simulink model "cart_pend_simulation"  (R2020a)
settings: Solver=VariableStepAuto  StartTime=0.0  StopTime=150  RelTol=1e-3
values from neighbouring files (symbols this model uses):
  a = 1/(M+m)    (= 0.1)    [cart_pend_script.m]
  A1 = [-1 max(z1) ... (first row only)    [TS_modling_script.m]    (also in cart_pend_script.m = [0 1 0 0; -17.31 0 0 0; 0 0 0 1; 1.7312 0 0 0])
  A2 = [-1 max(z1) ... (first row only)    [TS_modling_script.m]    (also in cart_pend_script.m = [0 1 0 0; -14.32 0 0 0; 0 0 0 1; 0.716 0 0 0])
  B1 = [0; -0.1765; 0; 0.1176]    [cart_pend_script.m]
  B2 = [0; -0.1147; 0; 0.1081]    [cart_pend_script.m]
  C = [1 0 0 0; 0 0 1 0; 0 0 0 1]    [cart_pend_script.m]
  g = 9.81    [cart_pend_script.m]
  Gl = [4 0 -1.5; -14.31 0 -6; 0 2 1; 1.73 0 4]    [cart_pend_script.m]
  Gnl = [0.1176 0 0; 0.3529 0 -0.1765; 0 0.1176 0; 0 0 0.1176]    [cart_pend_script.m]
  KK1 = lqr(Abf1,B1,Q,R,N)    [cart_pend_script.m]
  l = 0.5    [cart_pend_script.m]
  m = 2    [cart_pend_script.m]
  uc = 0.005    [cart_pend_script.m]
  x0 = [-0.7;1]    [TS_modling_script.m]    (also in cart_pend_script.m = [0.6; 0; 0.1; 0])
settings Model: Creator=pc  LastModifiedBy=hp
settings SolverCC: ZeroCrossAlgorithm=Adaptive
settings DebuggingCC: IgnoredZcDiagnostic=none

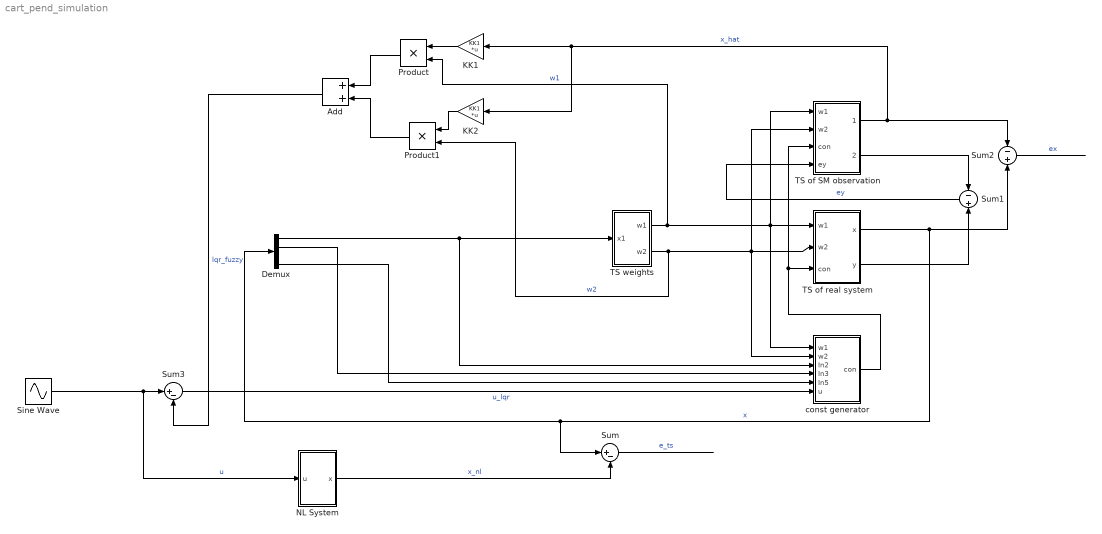
== system cart_pend_simulation ==
  Add : Sum
  Demux : Demux
  KK1 : Gain  Gain=KK1  Multiplication=Matrix(K*u)
  KK2 : Gain  Gain=KK1  Multiplication=Matrix(K*u)
  NL System : Subsystem
  Product : Product
  Product1 : Product
  Sine Wave : Sin  Amplitude=10  Frequency=5  SampleTime=0
  Sum : Sum  Inputs=|+-
  Sum1 : Sum  Inputs=-+
  Sum2 : Sum  Inputs=-+
  Sum3 : Sum  Inputs=|+-
  TS of SM observation : Subsystem
  TS of real system : Subsystem
  TS weights : Subsystem
  const generator : Subsystem
  wires:
  Demux/1 -> TS weights/1(x1), const generator/3(In2)
  TS weights/1(w1) -> Product/2, TS of SM observation/1(w1), const generator/1(w1), TS of real system/1(w1)  "w1"
  TS weights/2(w2) -> Product1/2, TS of SM observation/2(w2), const generator/2(w2), TS of real system/2(w2)  "w2"
  TS of real system/1(x) -> Sum/1, Demux/1, Sum2/2  "x"
  Demux/2 -> const generator/4(In3)
  Demux/4 -> const generator/5(In5)
  const generator/1(con) -> TS of SM observation/3(con), TS of real system/3(con)
  NL System/1(x) -> Sum/2  "x_nl"
  Sum/1 -> ?  "e_ts"
  Sum1/1 -> TS of SM observation/4(ey)  "ey"
  TS of SM observation/2(y_hat) -> Sum1/1
  TS of real system/2(y) -> Sum1/2
  TS of SM observation/1(x_hat) -> KK2/1, KK1/1, Sum2/1  "x_hat"
  Sum2/1 -> ?  "ex"
  Sine Wave/1 -> Sum3/1, NL System/1(u)  "u"
  Sum3/1 -> const generator/6(u)  "u_lqr"
  KK1/1 -> Product/1
  Product/1 -> Add/1
  KK2/1 -> Product1/1
  Product1/1 -> Add/2
  Add/1 -> Sum3/2  "lqr_fuzzy"

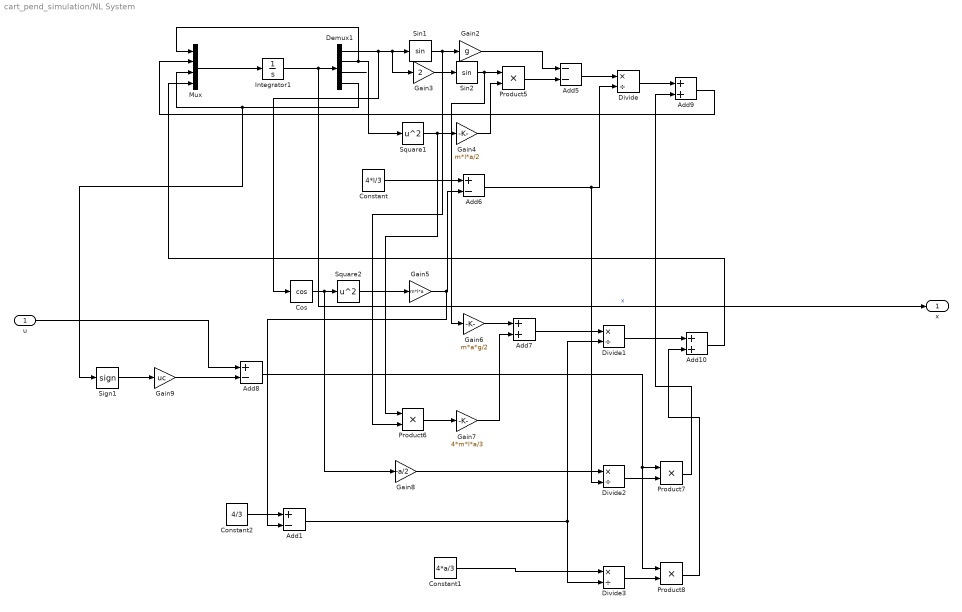
== system cart_pend_simulation/NL System ==
  u : Inport
  Add1 : Sum  Inputs=+-
  Add10 : Sum
  Add5 : Sum  Inputs=--
  Add6 : Sum  Inputs=+-
  Add7 : Sum
  Add8 : Sum  Inputs=+-
  Add9 : Sum
  Constant : Constant  Value=4*l/3
  Constant1 : Constant  Value=4*a/3
  Constant2 : Constant  Value=4/3
  Cos : Trigonometry  Operator=cos
  Demux1 : Demux
  Divide{,1..3} (4 alike) : Product  Inputs=*/
  Gain2 : Gain  Gain=g
  Gain3 : Gain  Gain=2
  Gain4 : Gain  Gain=m*l*a/2
  Gain5 : Gain  Gain=m*l*a
  Gain6 : Gain  Gain=m*a*g/2
  Gain7 : Gain  Gain=4*m*l*a/3
  Gain8 : Gain  Gain=-a/2
  Gain9 : Gain  Gain=uc
  Integrator1 : Integrator  InitialCondition=x0
  Mux : Mux
  Product{5..8} (4 alike) : Product
  Sign1 : Signum
  Sin1 : Trigonometry
  Sin2 : Trigonometry
  Square1 : Math  Operator=square  SaturateOnIntegerOverflow=on
  Square2 : Math  Operator=square  SaturateOnIntegerOverflow=on
  x : Outport
  wires:
  Add5/1 -> Divide/1
  Divide3/1 -> Product8/2
  Add9/1 -> Mux/2
  Add8/1 -> Product8/1, Product7/1
  Product5/1 -> Add5/2
  Square2/1 -> Gain5/1
  Demux1/4 -> Sign1/1, Mux/3
  Constant2/1 -> Add1/1
  Demux1/1 -> Cos/1, Gain3/1, Sin1/1
  Demux1/3 -> ?
  Add1/1 -> Divide1/2, Divide3/2
  Sin2/1 -> Gain6/1, Product5/1
  Add7/1 -> Divide1/1
  u/1 -> Add8/1
  Cos/1 -> Gain8/1, Square2/1
  Gain4/1 -> Product5/2
  Constant/1 -> Add6/1
  Divide1/1 -> Add10/1
  Gain5/1 -> Add1/2, Add6/2
  Gain9/1 -> Add8/2
  Product6/1 -> Gain7/1
  Divide2/1 -> Product7/2
  Gain8/1 -> Divide2/1
  Add6/1 -> Divide/2, Divide2/2
  Gain3/1 -> Sin2/1
  Sign1/1 -> Gain9/1
  Sin1/1 -> Product6/2, Gain2/1
  Square1/1 -> Product6/1, Gain4/1
  Gain2/1 -> Add5/1
  Product7/1 -> Add9/2
  Add10/1 -> Mux/4
  Product8/1 -> Add10/2
  Mux/1 -> Integrator1/1
  Demux1/2 -> Square1/1, Mux/1
  Gain7/1 -> Add7/2
  Integrator1/1 -> x/1, Demux1/1  "x"
  Divide/1 -> Add9/1
  Constant1/1 -> Divide3/1
  Gain6/1 -> Add7/1

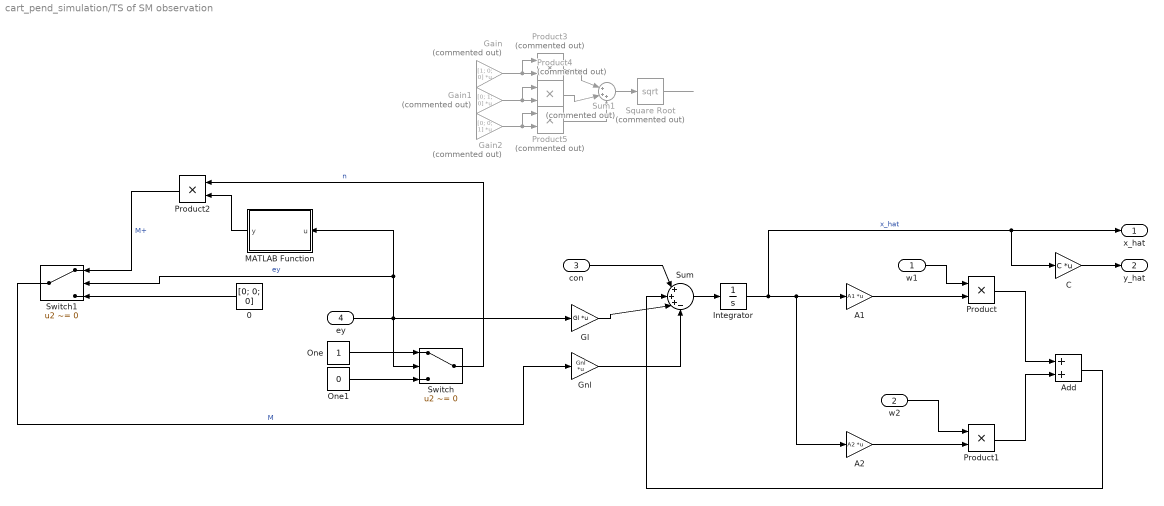
== system cart_pend_simulation/TS of SM observation ==
  w1 : Inport
  w2 : Inport  Port=2
  con : Inport  Port=3
  ey : Inport  Port=4
  0 : Constant  Value=[0; 0; 0]  VectorParams1D=off  OutDataTypeStr=Inherit: Inherit via back propagation
  A1 : Gain  Gain=A1  Multiplication=Matrix(K*u)
  A2 : Gain  Gain=A2  Multiplication=Matrix(K*u)
  Add : Sum
  C : Gain  Gain=C  Multiplication=Matrix(K*u)
  Gain : Gain  Commented=on  Gain=[1; 0; 0]  Multiplication=Matrix(K*u)
  Gain1 : Gain  Commented=on  Gain=[0; 1; 0]  Multiplication=Matrix(K*u)
  Gain2 : Gain  Commented=on  Gain=[0; 0; 1]  Multiplication=Matrix(K*u)
  Gl : Gain  Gain=Gl  Multiplication=Matrix(K*u)
  Gnl : Gain  Gain=Gnl  Multiplication=Matrix(K*u)
  Integrator : Integrator  InitialCondition=[0; 0; 0; 0]
  MATLAB Function : MATLAB Function  TreatAsAtomicUnit=on
  One : Constant  OutDataTypeStr=Inherit: Inherit via back propagation
  One1 : Constant  Value=0  OutDataTypeStr=Inherit: Inherit via back propagation
  Product : Product
  Product1 : Product
  Product2 : Product
  Product3 : Product  Commented=on
  Product4 : Product  Commented=on
  Product5 : Product  Commented=on
  Square Root : Sqrt  Commented=on  SaturateOnIntegerOverflow=on
  Sum : Sum  Inputs=|+++-
  Sum1 : Sum  Commented=on  Inputs=|+++
  Switch : Switch  Criteria=u2 ~= 0  ZeroCross=off
  Switch1 : Switch  Criteria=u2 ~= 0  ZeroCross=off
  x_hat : Outport
  y_hat : Outport  Port=2
  wires:
  Product/1 -> Add/1
  Integrator/1 -> C/1, x_hat/1, A2/1, A1/1  "x_hat"
  Add/1 -> Sum/2
  Sum/1 -> Integrator/1
  A1/1 -> Product/2
  A2/1 -> Product1/2
  Product1/1 -> Add/2
  w2/1 -> Product1/1
  w1/1 -> Product/1
  ey/1 -> Switch/2, Switch1/2, MATLAB Function/1(u), Gl/1  "ey"
  Gl/1 -> Sum/3
  Gnl/1 -> Sum/4
  C/1 -> y_hat/1
  One/1 -> Switch/1
  One1/1 -> Switch/3
  Switch1/1 -> Gnl/1  "M"
  MATLAB Function/1(y) -> Product2/2
  con/1 -> Sum/1
  Gain/1 -> Product3/1, Product3/2
  Gain1/1 -> Product4/1, Product4/2
  Gain2/1 -> Product5/1, Product5/2
  Product3/1 -> Sum1/1
  Product4/1 -> Sum1/2
  Product5/1 -> Sum1/3
  Sum1/1 -> Square Root/1
  Square Root/1 -> ?
  0/1 -> Switch1/3
  Product2/1 -> Switch1/1  "M+"
  Switch/1 -> Product2/1  "n"

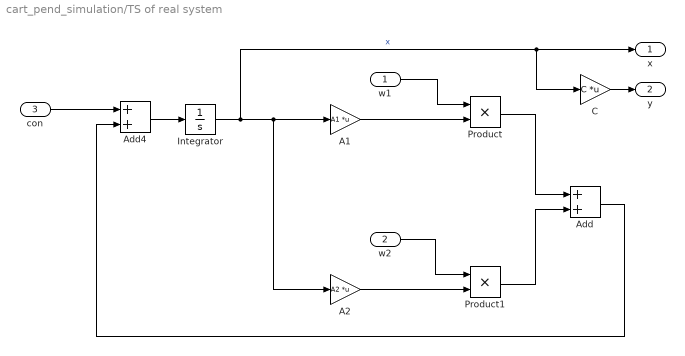
== system cart_pend_simulation/TS of real system ==
  w1 : Inport
  w2 : Inport  Port=2
  con : Inport  Port=3
  A1 : Gain  Gain=A1  Multiplication=Matrix(K*u)
  A2 : Gain  Gain=A2  Multiplication=Matrix(K*u)
  Add : Sum
  Add4 : Sum
  C : Gain  Gain=C  Multiplication=Matrix(K*u)
  Integrator : Integrator  InitialCondition=x0
  Product : Product
  Product1 : Product
  x : Outport
  y : Outport  Port=2
  wires:
  Product/1 -> Add/1
  Integrator/1 -> C/1, x/1, A2/1, A1/1  "x"
  con/1 -> Add4/1
  Add/1 -> Add4/2
  Add4/1 -> Integrator/1
  A1/1 -> Product/2
  A2/1 -> Product1/2
  Product1/1 -> Add/2
  w2/1 -> Product1/1
  w1/1 -> Product/1
  C/1 -> y/1

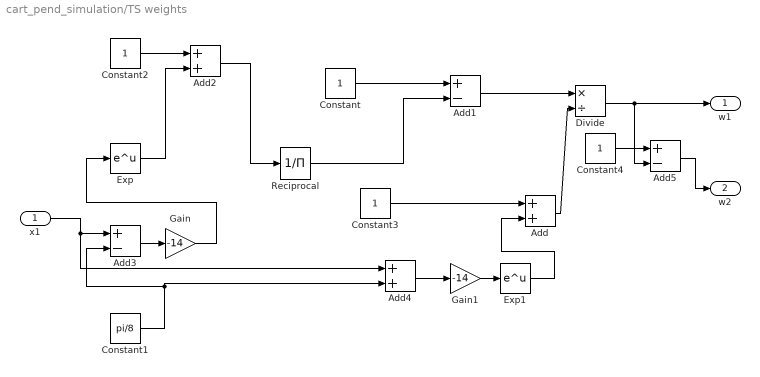
== system cart_pend_simulation/TS weights ==
  x1 : Inport
  Add : Sum
  Add1 : Sum  Inputs=+-
  Add2 : Sum
  Add3 : Sum  Inputs=+-
  Add4 : Sum
  Add5 : Sum  Inputs=+-
  Constant{,2..4} (4 alike) : Constant
  Constant1 : Constant  Value=pi/8
  Divide : Product  Inputs=*/
  Exp : Math  SaturateOnIntegerOverflow=on
  Exp1 : Math  SaturateOnIntegerOverflow=on
  Gain : Gain  Gain=-14
  Gain1 : Gain  Gain=-14
  Reciprocal : Product  Inputs=/  RndMeth=Zero  SaturateOnIntegerOverflow=on
  w1 : Outport
  w2 : Outport  Port=2
  wires:
  Reciprocal/1 -> Add1/2
  Gain/1 -> Exp/1
  Constant/1 -> Add1/1
  Constant2/1 -> Add2/1
  Add2/1 -> Reciprocal/1
  Add3/1 -> Gain/1
  Exp/1 -> Add2/2
  Constant1/1 -> Add4/2, Add3/2
  x1/1 -> Add4/1, Add3/1
  Add1/1 -> Divide/1
  Divide/1 -> Add5/2, w1/1
  Constant3/1 -> Add/1
  Add4/1 -> Gain1/1
  Gain1/1 -> Exp1/1
  Exp1/1 -> Add/2
  Add/1 -> Divide/2
  Constant4/1 -> Add5/1
  Add5/1 -> w2/1

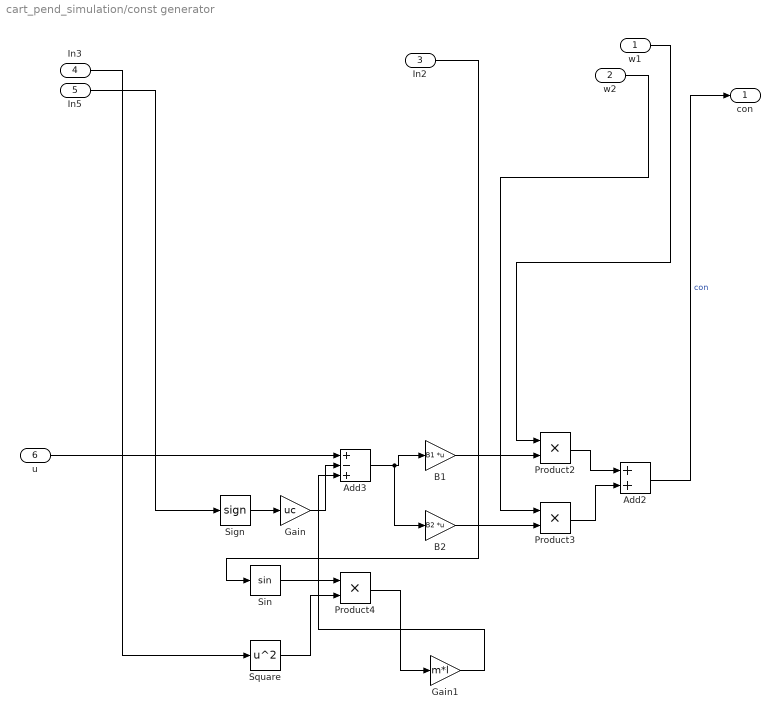
== system cart_pend_simulation/const generator ==
  w1 : Inport
  w2 : Inport  Port=2
  In2 : Inport  Port=3
  In3 : Inport  Port=4
  In5 : Inport  Port=5
  u : Inport  Port=6
  Add2 : Sum
  Add3 : Sum  Inputs=+-+
  B1 : Gain  Gain=B1  Multiplication=Matrix(K*u)
  B2 : Gain  Gain=B2  Multiplication=Matrix(K*u)
  Gain : Gain  Gain=uc
  Gain1 : Gain  Gain=m*l
  Product2 : Product
  Product3 : Product
  Product4 : Product
  Sign : Signum
  Sin : Trigonometry
  Square : Math  Operator=square  SaturateOnIntegerOverflow=on
  con : Outport
  wires:
  B1/1 -> Product2/2
  Gain1/1 -> Add3/3
  In2/1 -> Sin/1
  Product3/1 -> Add2/2
  Product4/1 -> Gain1/1
  Add3/1 -> B2/1, B1/1
  B2/1 -> Product3/2
  Product2/1 -> Add2/1
  Sign/1 -> Gain/1
  Square/1 -> Product4/2
  Gain/1 -> Add3/2
  Sin/1 -> Product4/1
  u/1 -> Add3/1
  Add2/1 -> con/1  "con"
  w2/1 -> Product3/1
  w1/1 -> Product2/1
  In3/1 -> Square/1
  In5/1 -> Sign/1

== matlab function cart_pend_simulation/TS of SM observation/MATLAB Function ==
  data: u input; y output
function y = fcn(u)
    
    P2 = [0.5 0 0; 0 0.25 0; 0 0 0.125];

y = -norm(P2)*inv(P2)*u/norm(u)
